simulink model "erfan_2"  (R2018b)
settings: Solver=VariableStepAuto  StartTime=0.0  StopTime=10.0  RelTol=1e-3
values from neighbouring files (symbols this model uses):
  Ct = double( subs( Ct) )    [main_sys.m]    (also in main_sys_klm.m; main_tf_10.m; main_tf_11.m; main_tf_12.m)
  K = P*C'/(C*P*C' + R)    [KALMAN.m]    (also in main_tf_9.m = lqi(sys_lq,Q,R))
  sys_sys = ss(A,B,C,D)    [main_sys.m]    (also in main_sys_klm.m; main_tf_10.m; main_tf_11.m; main_tf_12.m = ss(A_sys,B_sys,C_sys_mod,D_sys_mod))
undefined symbols (not defined in the file or in its folder): Continuous, Time
libraries: ctrlSharedLib x1
settings Model: Creator=eshojaei  LastModifiedBy=eshojaei

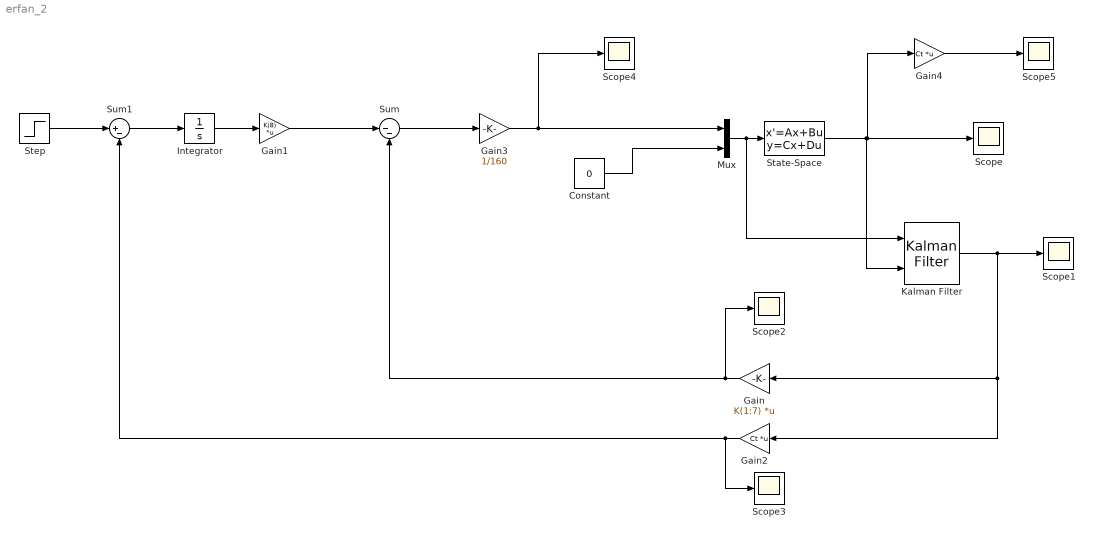
== system erfan_2 ==
  Constant : Constant  Value=0
  Gain : Gain  Gain=K(1:7)  Multiplication=Matrix(K*u)
  Gain1 : Gain  Gain=K(8)  Multiplication=Matrix(K*u)
  Gain2 : Gain  Gain=Ct  Multiplication=Matrix(K*u)
  Gain3 : Gain  Gain=1/160
  Gain4 : Gain  Gain=Ct  Multiplication=Matrix(K*u)
  Integrator : Integrator
  Kalman Filter : ctrlSharedLib/Kalman Filter  TimeDomain=Continuous-Time  UseCurrentEstimator=on  ModelSource=LTI State-Space Variable  ModelSourceVariable=sys_sys  A=0.95  B=1  C=1  D=0  NumberOfStates=1  NumberOfInputs=1  NumberOfOutputs=1  InitialEstimateSource=Dialog  X0=0  P0=10  UseK=off  UseGH=off  NumberOfProcessNoiseInputs=1  G=1  TimeInvariantG=on  H=0  TimeInvariantH=on  Q=0.05  TimeInvariantQ=on  R=1  TimeInvariantR=on  N=0  TimeInvariantN=on  AddInputPort=on  AddEnablePort=off  OutputEstimatedY=off  OutputP=off  Ts=-1
      settings: SourceProductBaseCode=CT
  Mux : Mux  Inputs=2
  Scope{,1..5} (6 alike) : Scope
  State-Space : StateSpace  A=sys_sys.A  B=sys_sys.B  C=sys_sys.C  D=sys_sys.D  InitialCondition=0
  Step : Step  Time=.1  After=10  SampleTime=0
  Sum : Sum  Inputs=|--
  Sum1 : Sum  Inputs=|+-
  wires:
  Mux/1 -> Kalman Filter/1, State-Space/1
  State-Space/1 -> Kalman Filter/2, Gain4/1, Scope/1
  Constant/1 -> Mux/2
  Kalman Filter/1 -> Gain2/1, Gain/1, Scope1/1
  Gain/1 -> Sum/2, Scope2/1
  Sum/1 -> Gain3/1
  Integrator/1 -> Gain1/1
  Gain1/1 -> Sum/1
  Sum1/1 -> Integrator/1
  Step/1 -> Sum1/1
  Gain2/1 -> Sum1/2, Scope3/1
  Gain3/1 -> Scope4/1, Mux/1
  Gain4/1 -> Scope5/1
